simulink model "Traction_Control"  (R2024a)
settings: Solver=VariableStepAuto  StartTime=0.0  StopTime=10.0  RelTol=1e-3
libraries: stmutilitieslib x2
settings Model: Creator=ezeki  LastModifiedBy=ezeki

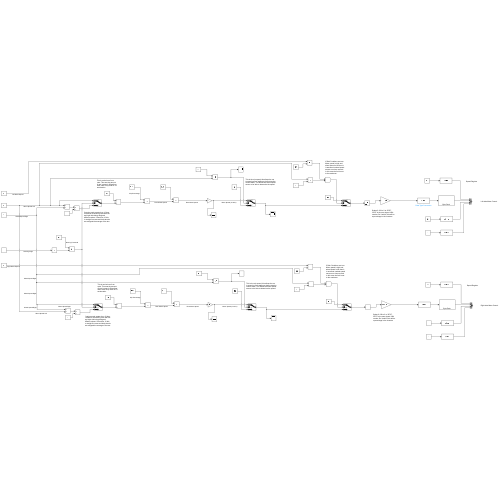
[thumbnail: Simulink's stored preview of the top-level diagram]
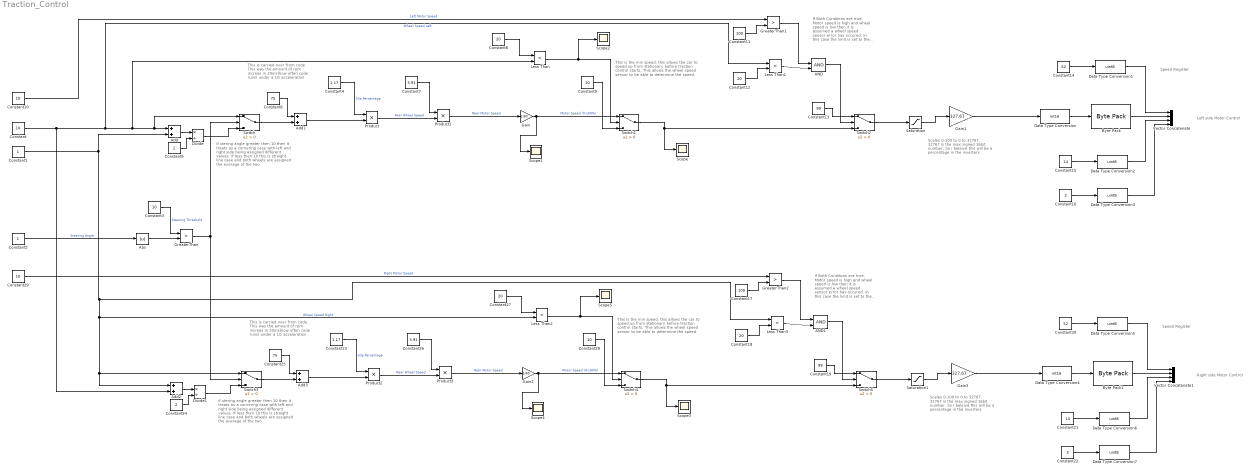
== system Traction_Control ==
  note: Left side Motor Control
  note: Speed Register
  note: Scales 0-100 to 0 to 32767, 32767 is the max signed 16bit number, So i beleive this will be a percentage in the inverters
  note: If Both Conditons are true. Motor speed is high and wheel speed is low then it is assumed a wheel speed sensor error has occured. In this case the limit is set to the maximum.
  note: This is the min speed, this allows the car to speed up from stationary before traction control starts, This allows the wheel speed sensor to be able to determine the speed.
  note: This is carried over from code. This was the amount of rpm increas in 20ms(how often code runs) under a 1G acceleration
  note: if stering angle greater then 10 then it treats as a cornering case with left and right side being assigned different values. If less then 10 this is straight line case and both wheels are assigned the average of the two.
  note: This is the min speed, this allows the car to speed up from stationary before traction control starts, This allows the wheel speed sensor to be able to determine the speed.
  note: Scales 0-100 to 0 to 32767, 32767 is the max signed 16bit number, So i beleive this will be a percentage in the inverters
  note: If Both Conditons are true. Motor speed is high and wheel speed is low then it is assumed a wheel speed sensor error has occured. In this case the limit is set to the maximum.
  note: This is carried over from code. This was the amount of rpm increas in 20ms(how often code runs) under a 1G acceleration
  note: Speed Register
  note: if stering angle greater then 10 then it treats as a cornering case with left and right side being assigned different values. If less then 10 this is straight line case and both wheels are assigned the average of the two.
  note: Right side Motor Control
  AND : Logic  IconShape=distinctive  AllPortsSameDT=off  OutDataTypeStr=boolean
  AND1 : Logic  IconShape=distinctive  AllPortsSameDT=off  OutDataTypeStr=boolean
  Abs : Abs  SaturateOnIntegerOverflow=off
  Add{,1..3} (4 alike) : Sum
  Byte Pack : stmutilitieslib/Byte Pack  datatypes={'int16'}  byteAlign=1  blockPlatform=stm32f4discovery
  Byte Pack1 : stmutilitieslib/Byte Pack  datatypes={'int16'}  byteAlign=1  blockPlatform=stm32f4discovery
  Constant{,3,9..10,28..29} (6 alike) : Constant  Value=10
  Constant1 : Constant
  Constant11 : Constant  Value=100
  Constant{8,12,18,27} (4 alike) : Constant  Value=20
  Constant13 : Constant  Value=99
  Constant14 : Constant  Value=52
  Constant15 : Constant  Value=14
  Constant16 : Constant  Value=3
  Constant17 : Constant  Value=100
  Constant19 : Constant  Value=99
  Constant2 : Constant
  Constant20 : Constant  Value=52
  Constant21 : Constant  Value=14
  Constant22 : Constant  Value=3
  Constant23 : Constant  Value=1.17
  Constant24 : Constant  Value=2
  Constant25 : Constant  Value=75
  Constant26 : Constant  Value=3.91
  Constant4 : Constant  Value=1.17
  Constant5 : Constant  Value=2
  Constant6 : Constant  Value=75
  Constant7 : Constant  Value=3.91
  Data Type Conversion : DataTypeConversion  OutDataTypeStr=int16  SaturateOnIntegerOverflow=off  RndMeth=Floor
  Data Type Conversion{1..3,5..7} (6 alike) : DataTypeConversion  OutDataTypeStr=uint8  SaturateOnIntegerOverflow=off  RndMeth=Floor
  Data Type Conversion4 : DataTypeConversion  OutDataTypeStr=int16  SaturateOnIntegerOverflow=off  RndMeth=Floor
  Divide : Product  Inputs=*/
  Divide1 : Product  Inputs=*/
  Gain : Gain  Gain=1/60
  Gain1 : Gain  Gain=327.67
  Gain2 : Gain  Gain=1/60
  Gain3 : Gain  Gain=327.67
  GreaterThan : RelationalOperator  Operator=>  OutDataTypeStr=boolean  RndMeth=Simplest  InputSameDT=off
  GreaterThan1 : RelationalOperator  Operator=>  OutDataTypeStr=boolean  RndMeth=Simplest  InputSameDT=off
  GreaterThan2 : RelationalOperator  Operator=>  OutDataTypeStr=boolean  RndMeth=Simplest  InputSameDT=off
  Less Than{,1..3} (4 alike) : RelationalOperator  Operator=<  OutDataTypeStr=boolean  RndMeth=Simplest  InputSameDT=off
  Product{,1..3} (4 alike) : Product
  Saturation : Saturate  UpperLimit=99  LowerLimit=0
  Saturation1 : Saturate  UpperLimit=99  LowerLimit=0
  Scope{,1..5} (6 alike) : Scope
  Switch{,1..5} (6 alike) : Switch  Criteria=u2 > Threshold  SaturateOnIntegerOverflow=off  InputSameDT=off
  Vector Concatenate : Concatenate  NumInputs=4
  Vector Concatenate1 : Concatenate  NumInputs=4
  wires:
  Constant2/1 -> Abs/1  "Steering Angle"
  Abs/1 -> GreaterThan/2
  Constant3/1 -> GreaterThan/1  "Steering Threshold"
  Add1/1 -> Product/2
  Constant4/1 -> Product/1  "Slip Percentage"
  Add/1 -> Divide/1
  Constant5/1 -> Divide/2
  Divide/1 -> Switch/3
  Switch/1 -> Add1/2
  Constant6/1 -> Add1/1
  Product/1 -> Product1/2  "Rear Wheel Speed"
  Constant7/1 -> Product1/1
  Product1/1 -> Gain/1  "Rear Motor Speed"
  Gain/1 -> Switch1/1, Scope1/1  "Motor Speed (0-100%)"
  Constant8/1 -> Less Than/1
  Less Than/1 -> Switch1/2, Scope2/1
  Constant9/1 -> Switch1/3
  Switch1/1 -> Switch2/3, Scope/1
  AND/1 -> Switch2/2
  Constant10/1 -> GreaterThan1/1  "Left Motor Speed"
  Constant11/1 -> GreaterThan1/2
  GreaterThan1/1 -> AND/1
  Constant12/1 -> Less Than1/2
  Less Than1/1 -> AND/2
  Constant13/1 -> Switch2/1
  Switch2/1 -> Saturation/1
  Saturation/1 -> Gain1/1
  Gain1/1 -> Data Type Conversion/1
  Data Type Conversion/1 -> Byte Pack/1
  Byte Pack/1 -> Vector Concatenate/2
  Constant14/1 -> Data Type Conversion1/1
  Data Type Conversion1/1 -> Vector Concatenate/1
  Data Type Conversion2/1 -> Vector Concatenate/3
  Constant15/1 -> Data Type Conversion2/1
  Data Type Conversion3/1 -> Vector Concatenate/4
  Constant16/1 -> Data Type Conversion3/1
  Data Type Conversion7/1 -> Vector Concatenate1/4
  Byte Pack1/1 -> Vector Concatenate1/2
  Data Type Conversion4/1 -> Byte Pack1/1
  Switch5/1 -> Saturation1/1
  Less Than3/1 -> AND1/2
  Gain3/1 -> Data Type Conversion4/1
  Constant19/1 -> Switch5/1
  Data Type Conversion5/1 -> Vector Concatenate1/1
  AND1/1 -> Switch5/2
  Switch4/1 -> Switch5/3, Scope3/1
  Data Type Conversion6/1 -> Vector Concatenate1/3
  GreaterThan2/1 -> AND1/1
  Constant27/1 -> Less Than2/1
  Constant17/1 -> GreaterThan2/2
  Constant29/1 -> GreaterThan2/1  "Right Motor Speed"
  Saturation1/1 -> Gain3/1
  Less Than2/1 -> Switch4/2, Scope5/1
  Gain2/1 -> Switch4/1, Scope4/1  "Motor Speed (0-100%)"
  Constant22/1 -> Data Type Conversion7/1
  Product3/1 -> Gain2/1  "Rear Motor Speed"
  Divide1/1 -> Switch3/3
  Constant21/1 -> Data Type Conversion6/1
  Add3/1 -> Product2/2
  Constant28/1 -> Switch4/3
  Add2/1 -> Divide1/1
  Constant23/1 -> Product2/1  "Slip Percentage"
  Product2/1 -> Product3/2  "Rear Wheel Speed"
  Constant18/1 -> Less Than3/2
  Constant24/1 -> Divide1/2
  Constant26/1 -> Product3/1
  Switch3/1 -> Add3/2
  Constant/1 -> Add2/2, Less Than1/1, Less Than/2, Switch/1, Add/1  "Wheel Speed Left"
  GreaterThan/1 -> Switch3/2, Switch/2
  Constant1/1 -> Add/2, Less Than2/2, Add2/1, Switch3/1, Less Than3/1  "Wheel Speed Right"
  Constant25/1 -> Add3/1
  Constant20/1 -> Data Type Conversion5/1
